simulink model "Project_r2022b"  (R2022b)
settings: Solver=VariableStepAuto  StartTime=0.0  StopTime=10.0  RelTol=1e-3
libraries: SignalEditorBlockLib x1
settings Model: Creator=mugiw  LastModifiedBy=mugiw
settings OptimizationCC: ReuseModelBlockBuffer=on
settings RTWCC: GPUComputeCapability=5.0

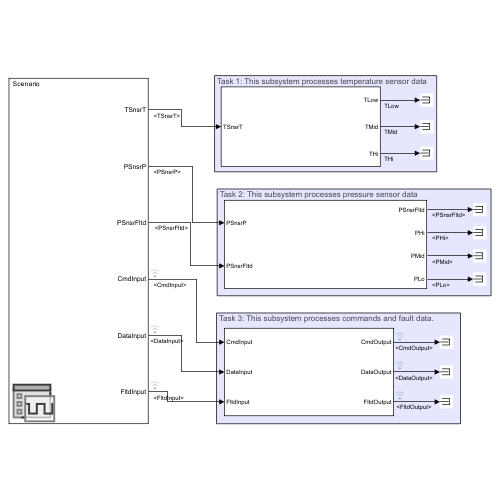
[thumbnail: Simulink's stored preview of the top-level diagram]
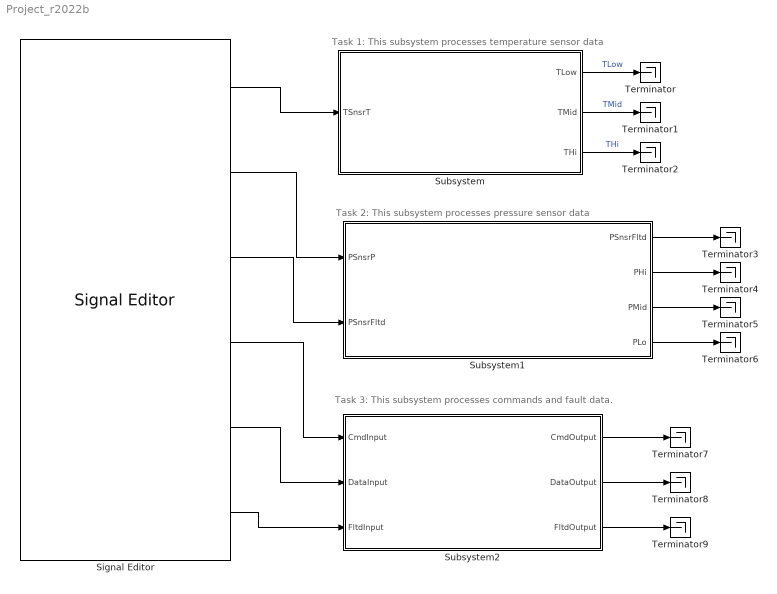
== system Project_r2022b ==
  note: Task 3: This subsystem processes commands and fault data.
  note: Task 2: This subsystem processes pressure sensor data
  note: Task 1: This subsystem processes temperature sensor data
  Signal Editor : SignalEditorBlockLib/Signal Editor  FileName=TempSignal.mat  ActiveScenario=Scenario  ActiveSignal=CmdInput  IsBus=off  OutputBusObjectStr=Bus: BusObject  SampleTime=0  Interpolate=off  ZeroCross=off  OutputAfterFinalValue=Setting to zero  Unit=inherit  PreserveSignalName=on
  Subsystem : Subsystem
  Subsystem1 : Subsystem
  Subsystem2 : Subsystem
  Terminator{,1..9} (10 alike) : Terminator
  wires:
  Subsystem/2(TMid) -> Terminator1/1  "TMid"
  Subsystem/3(THi) -> Terminator2/1  "THi"
  Subsystem/1(TLow) -> Terminator/1  "TLow"
  Subsystem1/1(PSnsrFltd) -> Terminator3/1
  Subsystem1/2(PHi) -> Terminator4/1
  Subsystem1/3(PMid) -> Terminator5/1
  Subsystem1/4(PLo) -> Terminator6/1
  Signal Editor/2 -> Subsystem1/1(PSnsrP)
  Signal Editor/1 -> Subsystem/1(TSnsrT)
  Signal Editor/3 -> Subsystem1/2("PSnsrFltd ")
  Signal Editor/4 -> Subsystem2/1(CmdInput)
  Signal Editor/5 -> Subsystem2/2(DataInput)
  Signal Editor/6 -> Subsystem2/3(FltdInput)
  Subsystem2/1(CmdOutput) -> Terminator7/1
  Subsystem2/2(DataOutput) -> Terminator8/1
  Subsystem2/3(FltdOutput) -> Terminator9/1

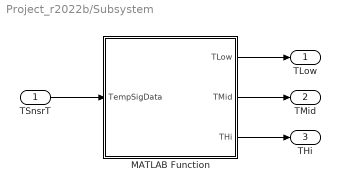
== system Project_r2022b/Subsystem ==
  TSnsrT : Inport
  MATLAB Function : MATLAB Function  TreatAsAtomicUnit=on
  TLow : Outport
  TMid : Outport  Port=2
  THi : Outport  Port=3
  wires:
  TSnsrT/1 -> MATLAB Function/1(TempSigData)
  MATLAB Function/1(TLow) -> TLow/1
  MATLAB Function/2(TMid) -> TMid/1
  MATLAB Function/3(THi) -> THi/1

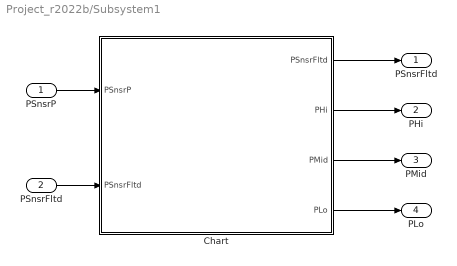
== system Project_r2022b/Subsystem1 ==
  PSnsrP : Inport
  "PSnsrFltd " : Inport  Port=2
  Chart : Stateflow chart  TreatAsAtomicUnit=on
  PSnsrFltd : Outport
  PHi : Outport  Port=2
  PMid : Outport  Port=3
  PLo : Outport  Port=4
  wires:
  Chart/1(PSnsrFltd) -> PSnsrFltd/1
  Chart/2(PHi) -> PHi/1
  Chart/3(PMid) -> PMid/1
  Chart/4(PLo) -> PLo/1
  "PSnsrFltd "/1 -> Chart/2("PSnsrFltd ")
  PSnsrP/1 -> Chart/1(PSnsrP)

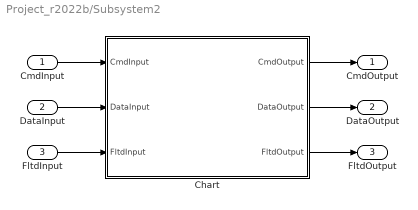
== system Project_r2022b/Subsystem2 ==
  CmdInput : Inport
  DataInput : Inport  Port=2
  FltdInput : Inport  Port=3
  Chart : Stateflow chart  TreatAsAtomicUnit=on
  CmdOutput : Outport
  DataOutput : Outport  Port=2
  FltdOutput : Outport  Port=3
  wires:
  FltdInput/1 -> Chart/3(FltdInput)
  DataInput/1 -> Chart/2(DataInput)
  CmdInput/1 -> Chart/1(CmdInput)
  Chart/1(CmdOutput) -> CmdOutput/1
  Chart/2(DataOutput) -> DataOutput/1
  Chart/3(FltdOutput) -> FltdOutput/1

== stateflow chart Project_r2022b/Subsystem1/Chart ==
  (default) -> (junction 57) : {PHi = false;
      | PMid = false;
      | PLo = false;}
  (junction 57) -> (junction 58) [order 1] : [PSnsrFltd == true]
  (junction 57) -> (junction 59) [order 2]
  (junction 58) -> (junction 66)
  (junction 59) -> (junction 60) [order 1] : [PSnsrP <= 100]
  (junction 59) -> (junction 61) [order 2]
  (junction 60) -> (junction 65) : {PLo = true;}
  (junction 61) -> (junction 62) [order 1] : [PSnsrP <= 200]
  (junction 61) -> (junction 63) [order 2] : {PHi = true;}
  (junction 62) -> (junction 64) : {PMid = true;}
  (junction 64) -> (junction 63)
  (junction 65) -> (junction 64)
  (junction 66) -> (junction 65)
  (junction 63) -> (junction 67)
  data: PSnsrP input; PSnsrFltd input; PSnsrFltd output; PHi output; PMid output; PLo output

== stateflow chart Project_r2022b/Subsystem2/Chart ==
  state Logic1
    entry:
    DataOutput = DataInput;
    CmdOutput = CmdInput;
    FltdOutput = FltdInput;
  state Logic2_3
    entry:
    DataOutput = 0;
    CmdOutput = false;
    FltdOutput = false;
  state Logic4
    entry:
    DataOutput = 0;
    CmdOutput = false;
    FltdOutput = true;
  Logic1 -> (junction 9) : [~CmdInput || FltdInput]
  (default) -> (junction 9)
  Logic2_3 -> (junction 9) : [CmdInput]
  (junction 9) -> Logic1 [order 1] : [CmdInput && ~FltdInput]
  (junction 9) -> Logic2_3 [order 2] : [~CmdInput]
  (junction 9) -> Logic4 [order 3] : %CmdInput && FltdInput
  Logic4 -> Logic2_3 : [~CmdInput]
  data: CmdInput input; DataInput input; FltdInput input; CmdOutput output; DataOutput output; FltdOutput output

== matlab function Project_r2022b/Subsystem/MATLAB Function ==
  data: TempSigData input; TLow output; TMid output; THi output
function [TLow,TMid,THi] = fcn(TempSigData)

TLow = false;
TMid = false;
THi = false;

if(TempSigData <= 100)
    TLow = true;
elseif((TempSigData > 100) && (TempSigData <= 200))
    TMid = true;
else
    THi = true;
end
